simulink model "Three_Ammeter_Method"  (R2021a)
settings: Solver=VariableStepAuto  StartTime=0.0  StopTime=0.05  RelTol=1e-3
libraries: spsCurrentMeasurementLib x3, spsRMSLib x3, spsSeriesRLCBranchLib x2, spsACVoltageSourceLib x1, spsGroundLib x1, spsPowerLib x1, spsVoltageMeasurementLib x1, spspowerguiLib x1
settings Model: Creator=tuhin  LastModifiedBy=tuhin

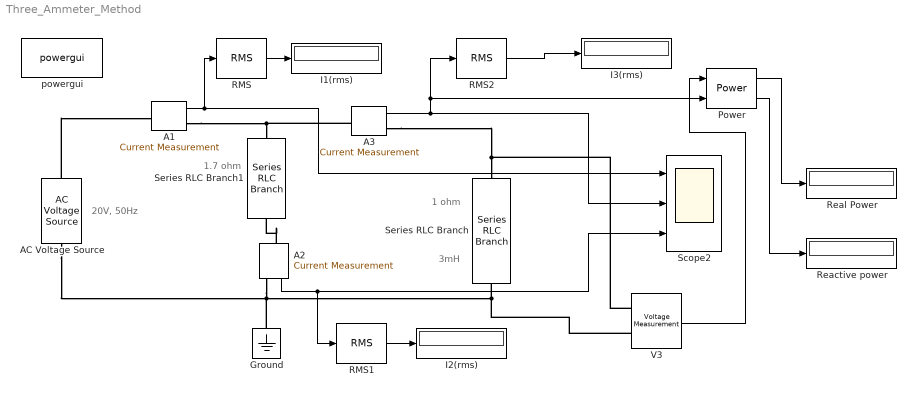
== system Three_Ammeter_Method ==
  note: 20V, 50Hz
  note: 3mH
  note: 1 ohm
  note: 1.7 ohm
  A1 : spsCurrentMeasurementLib/Current Measurement  PhasorSimulation=off  OutputType=Complex  PSBequivalent=0
  A2 : spsCurrentMeasurementLib/Current Measurement  PhasorSimulation=off  OutputType=Complex  PSBequivalent=0
  A3 : spsCurrentMeasurementLib/Current Measurement  PhasorSimulation=off  OutputType=Complex  PSBequivalent=0
  AC Voltage Source : spsACVoltageSourceLib/AC Voltage Source  Amplitude=28.28427125  Phase=0  Frequency=50  SampleTime=1e-6  Measurements=Voltage  BusType=swing  Pref=10e3  Qref=0  Qmin=-inf  Qmax=+inf
  Ground : spsGroundLib/Ground  LConnTagsString=a
  I1(rms) : Display
  I2(rms) : Display
  I3(rms) : Display
  Power : spsPowerLib/Power  Freq=60  Vinit=[1, 0]  Iinit=[1, 0]  Ts=0
      settings: SourceProductBaseCode=PS
  RMS : spsRMSLib/RMS  TrueRMS=on  Freq=60  RMSInit=120  Ts=0
  RMS1 : spsRMSLib/RMS  TrueRMS=on  Freq=60  RMSInit=120  Ts=0
  RMS2 : spsRMSLib/RMS  TrueRMS=on  Freq=60  RMSInit=120  Ts=0
  Reactive power : Display
  Real Power : Display
  Scope2 : Scope  NumInputPorts=3
  Series RLC Branch : spsSeriesRLCBranchLib/Series RLC Branch  LConnTagsString=__new0  RConnTagsString=__new0  BranchType=RL  Resistance=1  Inductance=3e-3  SetiL0=off  InitialCurrent=0  Capacitance=1e-6  Setx0=off  InitialVoltage=0  Measurements=None
  Series RLC Branch1 : spsSeriesRLCBranchLib/Series RLC Branch  LConnTagsString=__new0  RConnTagsString=__new0  BranchType=R  Resistance=1.7  Inductance=2e-3  SetiL0=off  InitialCurrent=0  Capacitance=1e-6  Setx0=off  InitialVoltage=0  Measurements=None
  V3 : spsVoltageMeasurementLib/Voltage Measurement  PhasorSimulation=off  OutputType=Complex  PSBequivalent=0
  powergui : spspowerguiLib/powergui  Priority=1  SimulationMode=Continuous  SampleTime=50e-6  frequency=60  Iterations=50  frequencyindice=50  Pbase=100e6  ErrMax=1e-4  UnitsV=kV  UnitsW=MW  buscounter=0  FunctionMessages=off  echomessages=off  EnableUseOfTLC=off  CurrentSourceSwitches=off  DisableSnubberDevices=off  DisableRonSwitches=off  DisableVfSwitches=off  DisplayEquations=off  AutomaticDiscreteSolvers=off  SolverType=Tustin/Backward Euler (TBE)  Interpol=off  ExternalGateDelay=off  methode=off  Ts=100  x0status=blocks  SPID=on  SwTol=0  HookPort=off  NonlinearTolerance=1e-4  nMaxIteration=100  ContinueOnMaxIteration=off  RestoreLinks=warning  ResistiveCurrentMeasurement=off  Frange=[0:2:500]  Ylog=off  Xlog=on  ShowGrid=off  save=off  variable=ZData  structure=0  ZoomFFT=off  StartTime=0.0  cycles=1  DisplayStyle=1  fundamental=60  FreqAxis=off  MaxFrequency=1000  frequencyindicesteady=1  RmsSteady=1  display=off
  wires:
  A1/1 -> RMS/1, Scope2/1
  A3/1 -> Power/2, RMS2/1, Scope2/2
  A2/1 -> RMS1/1, Scope2/3
  RMS2/1 -> I3(rms)/1
  RMS1/1 -> I2(rms)/1
  RMS/1 -> I1(rms)/1
  V3/1 -> Power/1
  Power/1 -> Real Power/1
  Power/2 -> Reactive power/1
  connections:
  AC Voltage Source/RConn1 -- A1/LConn1
  AC Voltage Source/LConn1 -- A2/RConn1 -- Ground/LConn1 -- V3/LConn2 -- Series RLC Branch/RConn1
  A3/RConn1 -- V3/LConn1 -- Series RLC Branch/LConn1
  A2/LConn1 -- Series RLC Branch1/RConn1
  A1/RConn1 -- A3/LConn1 -- Series RLC Branch1/LConn1
